simulink model "REALTIME_PART1_differentmethods"  (R2020b)
settings: Solver=FixedStepDiscrete  StartTime=0.0  StopTime=5  FixedStep=0.001  RelTol=1e-3
undefined symbols (not defined in the file or in its folder): den_Cz, National_Instruments, num_Cz, PCI, sens, step_size, T
libraries: sldrtlib x2
settings Model: ExtModeTrigDuration=6000  Creator=gioel  LastModifiedBy=pavarinlau
settings DataIOCC: ReturnWorkspaceOutputs=off
settings RTWCC: Description=Simulink Desktop Real-Time  SystemTargetFile=sldrt.tlc  TemplateMakefile=sldrt.tmf  RTWCompilerOptimization=on
settings CodeAppCC: MaxIdLength=95
settings SimulinkDesktopRealTimeCC: TargetPreCompLibLocation=C:\Program Files\MATLAB\R2020b\toolbox\sldrt\lib\win64

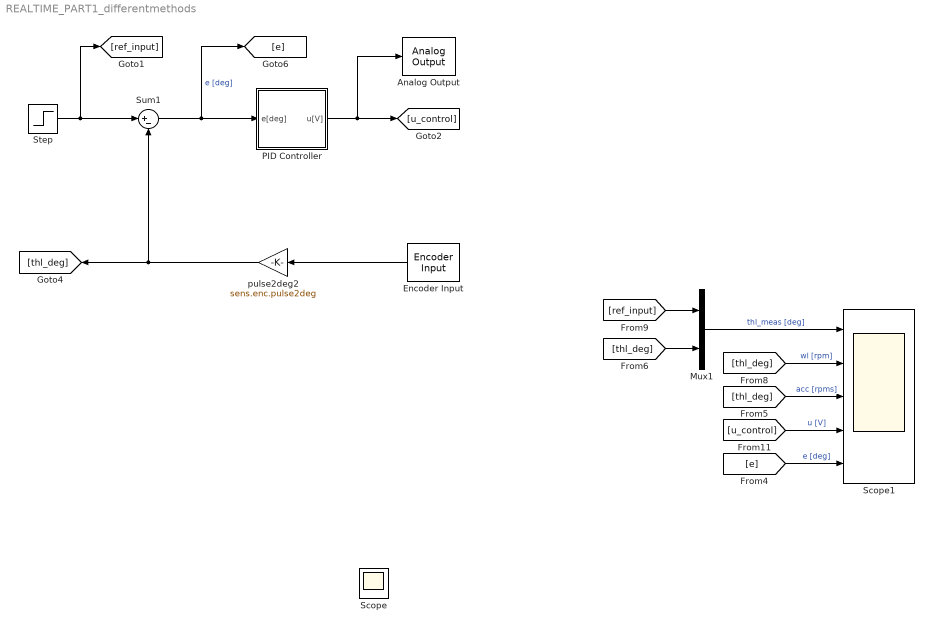
== system REALTIME_PART1_differentmethods ==
  Analog Output : sldrtlib/Analog Output  SampleTime=-1  MaxMissedTicks=10  ShowMissedTicks=off  YieldWhenWaiting=off  DrvName=National_Instruments/PCI-6221  DrvAddress=4294967295  DrvOptions=[0 0 0 2 0]  Channels=1  RangeMode=1  VoltRange=1  InitialValue=0  FinalValue=0
      settings: AttributesFormatString=National Instruments\nPCI-6221 [auto]
  Encoder Input : sldrtlib/Encoder Input  SampleTime=T  MaxMissedTicks=10  ShowMissedTicks=off  YieldWhenWaiting=off  DrvName=National_Instruments/PCI-6221  DrvAddress=4294967295  DrvOptions=[0 0 0 2 0]  Channels=1  QuadMode=3  IndexPulse=1  InputFilter=Inf  DataType=1
      settings: AttributesFormatString=National Instruments\nPCI-6221 [auto]
  Mux1 : Mux  Inputs=2
  PID Controller : Subsystem
  Scope1 : Scope  NumInputPorts=5
  Step : Step  After=step_size  SampleTime=T
  Sum1 : Sum  Inputs=|+-
  pulse2deg2 : Gain  Gain=sens.enc.pulse2deg
  Scope : Scope
  wires:
  Sum1/1 -> PID Controller/1(e[deg]), [e]  "e [deg]"
  Step/1 -> Sum1/1, [ref_input]
  PID Controller/1(u[V]) -> Analog Output/1, [u_control]
  Mux1/1 -> Scope1/1  "thl_meas [deg]"
  [thl_deg] -> Mux1/2
  [thl_deg] -> Scope1/3  "acc [rpms]"
  [thl_deg] -> Scope1/2  "wl [rpm]"
  [ref_input] -> Mux1/1
  pulse2deg2/1 -> Sum1/2, [thl_deg]
  Encoder Input/1 -> pulse2deg2/1
  [e] -> Scope1/5  "e [deg]"
  [u_control] -> Scope1/4  "u [V]"

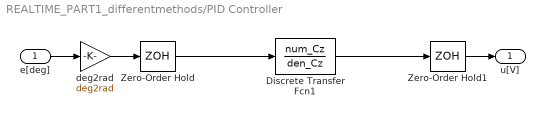
== system REALTIME_PART1_differentmethods/PID Controller ==
  e[deg] : Inport
  Discrete Transfer Fcn1 : DiscreteTransferFcn  Numerator=num_Cz  Denominator=den_Cz  SampleTime=T
  Zero-Order Hold : ZeroOrderHold  SampleTime=T
  Zero-Order Hold1 : ZeroOrderHold  SampleTime=T
  deg2rad : Gain  Gain=deg2rad
  u[V] : Outport
  wires:
  Discrete Transfer Fcn1/1 -> Zero-Order Hold1/1
  Zero-Order Hold/1 -> Discrete Transfer Fcn1/1
  deg2rad/1 -> Zero-Order Hold/1
  e[deg]/1 -> deg2rad/1
  Zero-Order Hold1/1 -> u[V]/1
